simulink model "julien"  (Simulink 7.4)
settings: Solver=FixedStepDiscrete  StartTime=0.0  StopTime=inf  FixedStep=0.01  RelTol=1e-3
PreLoadFcn:
  | RTWConfigurationCB('preloadfcn', bdroot);
PostLoadFcn:
  | mpc555rt_switch_target(gcs,'auto')
undefined symbols (not defined in the file or in its folder): integration01, integration02
libraries: mpc555drivers x5, NAV420Lib x3
CloseFcn:
  | rtwprivate ssgencode ModelCloseRequest foo
settings Model: Creator=The MathWorks Inc.  LastModifiedBy=autopilot
settings DataIOCC: SignalLoggingName=sigsOut
settings OptimizationCC: InlineParams=on  InlineInvariantSignals=on  EnforceIntegerDowncast=off  ZeroExternalMemoryAtStartup=off  ZeroInternalMemoryAtStartup=off  InitFltsAndDblsToZero=on  NoFixptDivByZeroProtection=on  OptimizeModelRefInitCode=on  LifeSpan=1
settings DebuggingCC: SaveWithParameterizedLinksMsg=none  SignalResolutionControl=TryResolveAllWithWarning  SolverPrmCheckMsg=none  MultiTaskDSMMsg=warning  MultiTaskCondExecSysMsg=none  UnderSpecifiedDataTypeMsg=error  StrictBusMsg=None
settings HardwareCC: ProdEndianess=BigEndian  ProdHWDeviceType=Motorola PowerPC
settings RTWCC: SystemTargetFile=mpc555rt.tlc  TemplateMakefile=mpc555rt.tmf  Description=Target Support Package (for use with Freescale MPC5xx) (real-time)  ProcessScript=mpc555rt_make_rtw_hook
settings CodeAppCC: IgnoreCustomStorageClasses=off
settings STFCustomTargetCC: TargetFcnLib=ansi_tfl_tmw.mat  TargetLibSuffix=.a  TargetPreCompLibLocation=C:\Program Files\MATLAB\R2009b\toolbox\rtw\targets\mpc555dk\drivers\lib\DIAB  IncludeMdlTerminateFcn=off  CombineOutputUpdateFcns=on  ERTCustomFileBanners=on  SupportAbsoluteTime=off  SupportNonFinite=off  SupportComplex=off  SupportContinuousTime=off  SupportNonInlinedSFcns=off  CPPClassGenCompliant=on  SystemTargetFile=mpc555rt.tlc
settings ERTTargetCC: TargetFcnLib=ansi_tfl_tmw.mat  TargetPreCompLibLocation=C:\Program Files\MATLAB\R2009b\toolbox\rtw\targets\mpc555dk\drivers\lib\DIAB  MultiwordLength=2048  ParMdlRefBuildCompliant=off  CompOptLevelCompliant=off  IncludeMdlTerminateFcn=off  ERTFirstTimeCompliant=off  SupportAbsoluteTime=off  SupportNonFinite=off  SupportComplex=off  ModelStepFunctionPrototypeControlCompliant=off  ExtModeMexFile=MPC5xxExternalModeOpen  ExtModeIntrfLevel=Level2 - Open  ERTCustomFileTemplate=example_file_process.tlc  ConvertIfToSwitch=off
settings CustomProperty: DataType=RTWOptions_EnumType__toolbox_rtw_targets_mpc555dk_mpc555dk_mpc555rt_1MPC555_OPTIMIZATION_SWITCH  Value=speed
settings EnumStrPairs: String=speed

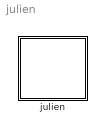
== system julien ==
  julien : Subsystem  InitFcn=|
      | % START RTW CONFIGURATION CODE %
      | RTWConfigurationCB('rtw_target_initfcn',gcb);
      | % END RTW CONFIGURATION CODE %
      mask Display: image(imread('target_affordance_icon.jpg'),'bottom-right')

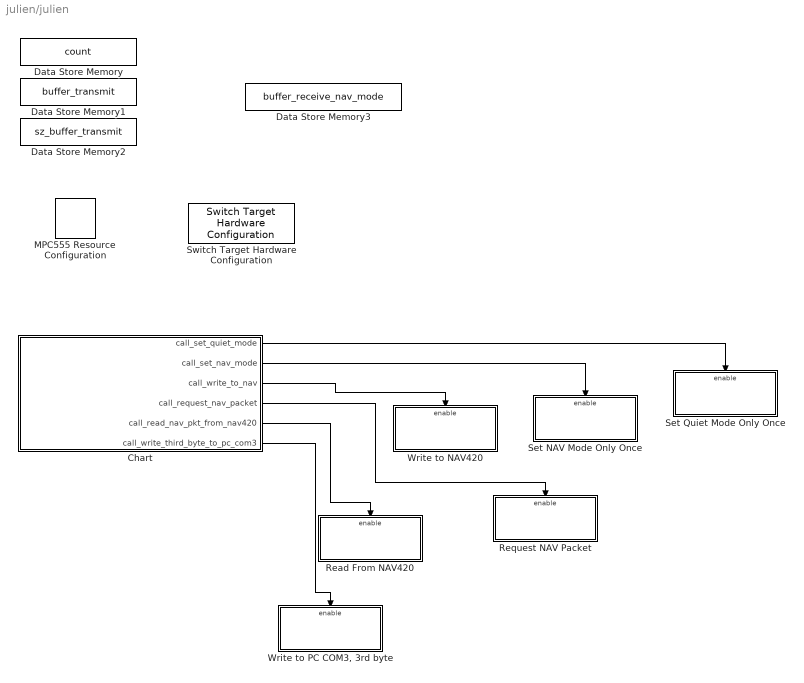
== system julien/julien ==
  Chart : Stateflow chart
  Data Store Memory : DataStoreMemory  DataStoreName=count  DataType=uint8  OutDataType=fixdt(1, 16)  OutScaling=2^0  OutDataTypeStr=uint8
  Data Store Memory1 : DataStoreMemory  DataStoreName=buffer_transmit  InitialValue=[0 0 0 0 0 0 0 0 0 0 0]  DataType=uint8  OutDataType=fixdt(1, 16)  OutScaling=2^0  OutDataTypeStr=uint8
  Data Store Memory2 : DataStoreMemory  DataStoreName=sz_buffer_transmit  DataType=uint32  OutDataType=fixdt(1, 16)  OutScaling=2^0  OutDataTypeStr=uint32
  Data Store Memory3 : DataStoreMemory  DataStoreName=buffer_receive_nav_mode  InitialValue=[0 0 0 0 0 0 0 0 0 0 0 0 0 0 0 0 0 0 0 0 0 0 0 0 0 0 0 0 0 0 0 0 0 0 0 0 0]  DataType=uint8  OutDataType=fixdt(1, 16)  OutScaling=2^0  OutDataTypeStr=uint8
  MPC555 Resource Configuration : mpc555drivers/MPC555 Resource Configuration  Tag=RTW CONFIGURATION BLOCK  Priority=-100000  SystemSampleTime=-1  oldParentName=integration02/integration01  oldBlockName=|  defaultConfigLibrary=mpc555drivers
      | integration02/integration01/MPC555
      | Resource
      | Configuration
  Read From NAV420 : Subsystem  TreatAsAtomicUnit=on
  Request NAV Packet : Subsystem  TreatAsAtomicUnit=on
  Set NAV Mode Only Once : Subsystem  TreatAsAtomicUnit=on
  Set Quiet Mode Only Once : Subsystem  TreatAsAtomicUnit=on
  Switch Target Hardware Configuration : mpc555drivers/Utilities/Switch Target Hardware Configuration  SystemSampleTime=-1
  Write to NAV420 : Subsystem  TreatAsAtomicUnit=on
  "Write to PC COM3, 3rd byte" : Subsystem  TreatAsAtomicUnit=on
  wires:
  Chart/2(call_set_nav_mode) -> Set NAV Mode Only Once/Enable
  Chart/3(call_write_to_nav) -> Write to NAV420/Enable
  Chart/4(call_request_nav_packet) -> Request NAV Packet/Enable
  Chart/1(call_set_quiet_mode) -> Set Quiet Mode Only Once/Enable
  Chart/5(call_read_nav_pkt_from_nav420) -> Read From NAV420/Enable
  Chart/6(call_write_third_byte_to_pc_com3) -> "Write to PC COM3, 3rd byte"/Enable

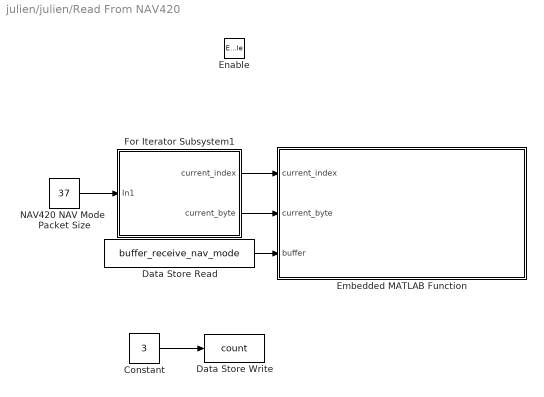
== system julien/julien/Read From NAV420 ==
  Enable : EnablePort
  Constant : Constant  Value=3  OutDataTypeMode=uint8  OutDataType=fixdt(1, 16)  OutScaling=2^0  OutDataTypeStr=uint8
  Data Store Read : DataStoreRead  DataStoreName=buffer_receive_nav_mode  SampleTime=-1
  Data Store Write : DataStoreWrite  DataStoreName=count  SampleTime=-1
  Embedded MATLAB Function : Stateflow chart
  For Iterator Subsystem1 : Subsystem  TreatAsAtomicUnit=on
  NAV420 NAV Mode  Packet Size : Constant  Value=37  OutDataType=fixdt(1, 16)  OutScaling=2^0
  wires:
  NAV420 NAV Mode  Packet Size/1 -> For Iterator Subsystem1/1(In1)
  Data Store Read/1 -> Embedded MATLAB Function/3(buffer)
  For Iterator Subsystem1/2(current_byte) -> Embedded MATLAB Function/2(current_byte)
  For Iterator Subsystem1/1(current_index) -> Embedded MATLAB Function/1(current_index)
  Constant/1 -> Data Store Write/1

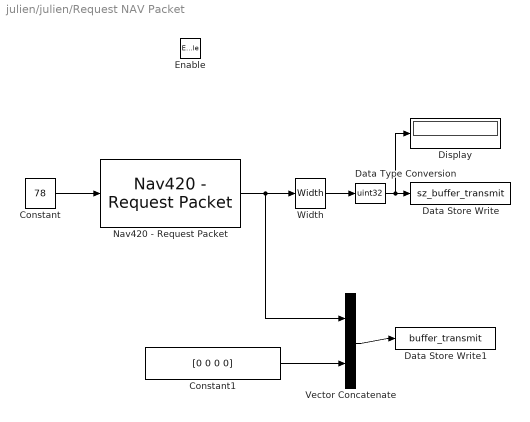
== system julien/julien/Request NAV Packet ==
  Enable : EnablePort
  Constant : Constant  Value=78  OutDataTypeMode=int8  OutDataType=fixdt(1, 16)  OutScaling=2^0  OutDataTypeStr=int8
  Constant1 : Constant  Value=[0 0 0 0]  OutDataTypeMode=uint8  OutDataType=fixdt(1, 16)  OutScaling=2^0  OutDataTypeStr=uint8
  Data Store Write : DataStoreWrite  DataStoreName=sz_buffer_transmit  SampleTime=-1
  Data Store Write1 : DataStoreWrite  DataStoreName=buffer_transmit  SampleTime=-1
  Data Type Conversion : DataTypeConversion  OutDataTypeMode=uint32  OutDataType=fixdt(1, 16)  OutScaling=2^0  OutDataTypeStr=uint32
  Display : Display
  Nav420 - Request Packet : NAV420Lib/Nav420 - Request Packet  SystemSampleTime=-1
  Vector Concatenate : Concatenate  Mode=Vector
  Width : Width
  wires:
  Constant/1 -> Nav420 - Request Packet/1
  Nav420 - Request Packet/1 -> Width/1, Vector Concatenate/1
  Width/1 -> Data Type Conversion/1
  Data Type Conversion/1 -> Data Store Write/1, Display/1
  Constant1/1 -> Vector Concatenate/2
  Vector Concatenate/1 -> Data Store Write1/1

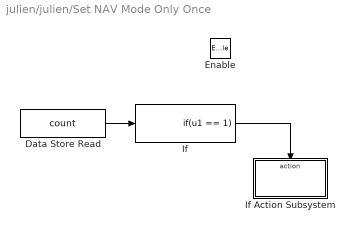
== system julien/julien/Set NAV Mode Only Once ==
  Enable : EnablePort
  Data Store Read : DataStoreRead  DataStoreName=count  SampleTime=-1
  If : If  IfExpression=u1 == 1  ShowElse=off
  If Action Subsystem : Subsystem  TreatAsAtomicUnit=on
  wires:
  Data Store Read/1 -> If/1
  If/1 -> If Action Subsystem/Action

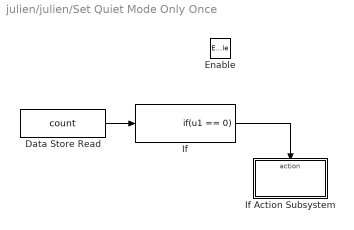
== system julien/julien/Set Quiet Mode Only Once ==
  Enable : EnablePort
  Data Store Read : DataStoreRead  DataStoreName=count  SampleTime=-1
  If : If  IfExpression=u1 == 0  ShowElse=off
  If Action Subsystem : Subsystem  TreatAsAtomicUnit=on
  wires:
  Data Store Read/1 -> If/1
  If/1 -> If Action Subsystem/Action

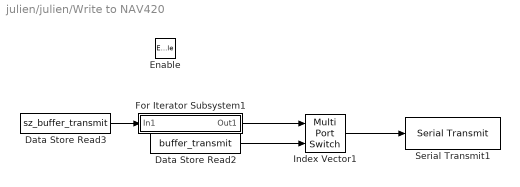
== system julien/julien/Write to NAV420 ==
  Enable : EnablePort
  Data Store Read2 : DataStoreRead  DataStoreName=buffer_transmit  SampleTime=-1
  Data Store Read3 : DataStoreRead  DataStoreName=sz_buffer_transmit  SampleTime=-1
  For Iterator Subsystem1 : Subsystem  TreatAsAtomicUnit=on
  Index Vector1 : MultiPortSwitch  Inputs=1  OutDataType=fixdt(1, 16)  OutScaling=2^0
  Serial Transmit1 : mpc555drivers/Serial Communications Interface (SCI)/Serial Transmit  module=2  show_length=off  show_num_sent=off  T=-1
  wires:
  Data Store Read3/1 -> For Iterator Subsystem1/1(In1)
  Data Store Read2/1 -> Index Vector1/2
  For Iterator Subsystem1/1(Out1) -> Index Vector1/1
  Index Vector1/1 -> Serial Transmit1/1

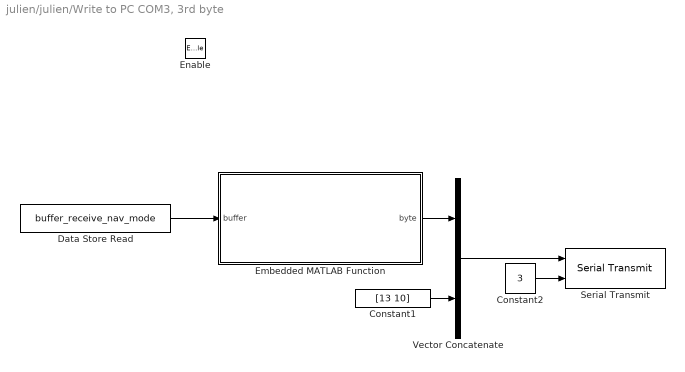
== system julien/julien/Write to PC COM3, 3rd byte ==
  Enable : EnablePort
  Constant1 : Constant  Value=[13 10]  OutDataTypeMode=uint8  OutDataType=fixdt(1, 16)  OutScaling=2^0  OutDataTypeStr=uint8
  Constant2 : Constant  Value=3  OutDataTypeMode=uint32  OutDataType=fixdt(1, 16)  OutScaling=2^0  OutDataTypeStr=uint32
  Data Store Read : DataStoreRead  DataStoreName=buffer_receive_nav_mode  SampleTime=-1
  Embedded MATLAB Function : Stateflow chart
  Serial Transmit : mpc555drivers/Serial Communications Interface (SCI)/Serial Transmit  module=1  show_length=on  show_num_sent=off  T=-1
  Vector Concatenate : Concatenate  Mode=Vector
  wires:
  Data Store Read/1 -> Embedded MATLAB Function/1(buffer)
  Embedded MATLAB Function/1(byte) -> Vector Concatenate/1
  Constant1/1 -> Vector Concatenate/2
  Vector Concatenate/1 -> Serial Transmit/1
  Constant2/1 -> Serial Transmit/2

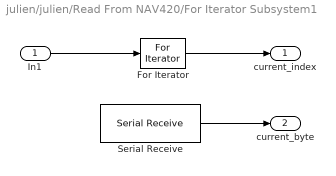
== system julien/julien/Read From NAV420/For Iterator Subsystem1 ==
  In1 : Inport  OutDataType=fixdt(1, 16)  OutScaling=2^0
  For Iterator : ForIterator  IterationSource=external
  Serial Receive : mpc555drivers/Serial Communications Interface (SCI)/Serial Receive  module=2  show_length=off  max_length=1  show_reset=off  show_bytes_read=off  show_flags=off  show_overrun=off  T=-1
  current_index : Outport  OutDataType=fixdt(1, 16)  OutScaling=2^0
  current_byte : Outport  Port=2  DataType=uint8  OutDataType=fixdt(1, 16)  OutScaling=2^0  OutDataTypeStr=uint8
  wires:
  In1/1 -> For Iterator/1
  For Iterator/1 -> current_index/1
  Serial Receive/1 -> current_byte/1

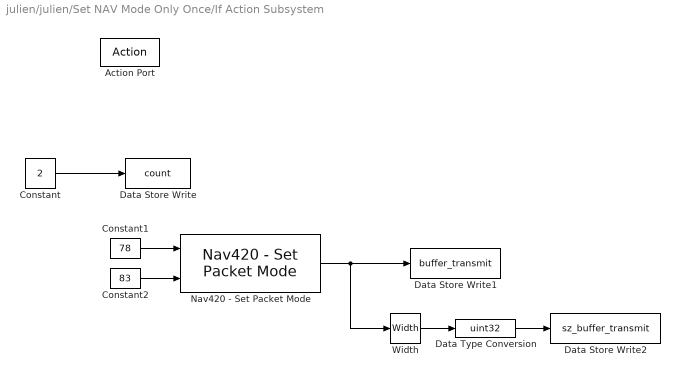
== system julien/julien/Set NAV Mode Only Once/If Action Subsystem ==
  Action Port : ActionPort  ActionType=then
  Constant : Constant  Value=2  OutDataTypeMode=uint8  OutDataType=fixdt(1, 16)  OutScaling=2^0  OutDataTypeStr=uint8  SampleTime=-1
  Constant1 : Constant  Value=78  OutDataTypeMode=int8  OutDataType=fixdt(1, 16)  OutScaling=2^0  OutDataTypeStr=int8  SampleTime=-1
  Constant2 : Constant  Value=83  OutDataTypeMode=int8  OutDataType=fixdt(1, 16)  OutScaling=2^0  OutDataTypeStr=int8  SampleTime=-1
  Data Store Write : DataStoreWrite  DataStoreName=count  SampleTime=-1
  Data Store Write1 : DataStoreWrite  DataStoreName=buffer_transmit  SampleTime=-1
  Data Store Write2 : DataStoreWrite  DataStoreName=sz_buffer_transmit  SampleTime=-1
  Data Type Conversion : DataTypeConversion  OutDataTypeMode=uint32  OutDataType=fixdt(1, 16)  OutScaling=2^0  OutDataTypeStr=uint32
  Nav420 - Set Packet Mode : NAV420Lib/Nav420 - Set Packet Mode  SystemSampleTime=-1
  Width : Width
  wires:
  Constant/1 -> Data Store Write/1
  Constant1/1 -> Nav420 - Set Packet Mode/1
  Constant2/1 -> Nav420 - Set Packet Mode/2
  Width/1 -> Data Type Conversion/1
  Data Type Conversion/1 -> Data Store Write2/1
  Nav420 - Set Packet Mode/1 -> Data Store Write1/1, Width/1

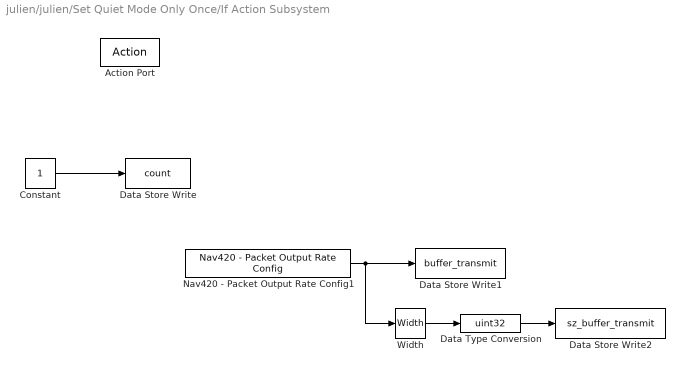
== system julien/julien/Set Quiet Mode Only Once/If Action Subsystem ==
  Action Port : ActionPort  ActionType=then
  Constant : Constant  OutDataTypeMode=uint8  OutDataType=fixdt(1, 16)  OutScaling=2^0  OutDataTypeStr=uint8  SampleTime=-1
  Data Store Write : DataStoreWrite  DataStoreName=count  SampleTime=-1
  Data Store Write1 : DataStoreWrite  DataStoreName=buffer_transmit  SampleTime=-1
  Data Store Write2 : DataStoreWrite  DataStoreName=sz_buffer_transmit  SampleTime=-1
  Data Type Conversion : DataTypeConversion  OutDataTypeMode=uint32  OutDataType=fixdt(1, 16)  OutScaling=2^0  OutDataTypeStr=uint32
  Nav420 - Packet Output Rate Config1 : NAV420Lib/Nav420 - Packet Output Rate Config  SystemSampleTime=-1  shouldSave=off  output_rate=0
  Width : Width
  wires:
  Constant/1 -> Data Store Write/1
  Nav420 - Packet Output Rate Config1/1 -> Data Store Write1/1, Width/1
  Width/1 -> Data Type Conversion/1
  Data Type Conversion/1 -> Data Store Write2/1

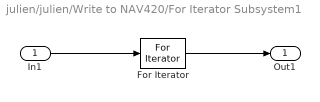
== system julien/julien/Write to NAV420/For Iterator Subsystem1 ==
  In1 : Inport  OutDataType=fixdt(1, 16)  OutScaling=2^0
  For Iterator : ForIterator  IterationSource=external
  Out1 : Outport  OutDataType=fixdt(1, 16)  OutScaling=2^0
  wires:
  In1/1 -> For Iterator/1
  For Iterator/1 -> Out1/1

== matlab function julien/Read From NAV420/Embedded MATLAB Function ==
  data: current_index input double; current_byte input double; buffer input double
function cat_nav_packet(current_index,current_byte,buffer)

%#eml


buffer( current_index ) = current_byte;

== stateflow chart julien/Chart ==
  state Step1
    count=0;
    call_set_quiet_mode=1;
    call_write_to_nav=1;
  state End
    call_request_nav_packet=1;
    call_write_to_nav=1;
    call_read_nav_pkt_from_nav420=1;
    call_write_third_byte_to_pc_com3=1;
  state Step2
    call_set_nav_mode=1;
    call_write_to_nav=1;
  (default) -> Step1
  Step1 -> Step2 : [count==1]
  Step2 -> End : [count==2]
  End -> End
  data: count data_store_memory double; call_set_quiet_mode output uint8; call_set_nav_mode output uint8; call_write_to_nav output uint8; call_request_nav_packet output uint8; call_read_nav_pkt_from_nav420 output uint8; call_write_third_byte_to_pc_com3 output uint8

== matlab function julien/Write to PC COM3, 3rd byte/Embedded MATLAB Function ==
  data: buffer input double; byte output double
function byte = extract_third_byte(buffer)

%#eml


byte = buffer( 3 );
